simulink model "CP_SFC_Lin_a_n9558292"  (R2018a)
settings: Solver=ode4  StartTime=0.0  StopTime=5  FixedStep=0.02  RelTol=1e-3
values from neighbouring files (symbols this model uses):
  g = 9.81    [CP_SFC_Lin_b_MainFile_n9558292.m]
  l = 0.2    [CP_SFC_Lin_b_MainFile_n9558292.m]
  m = 0.15    [CP_SFC_Lin_b_MainFile_n9558292.m]
  Mc = 0.4    [CP_SFC_Lin_b_MainFile_n9558292.m]
  x10 = 0.4    [CP_SFC_Lin_b_MainFile_n9558292.m]
  x20 = deg2rad(200)    [CP_SFC_Lin_b_MainFile_n9558292.m]
  x30 = 0    [CP_SFC_Lin_b_MainFile_n9558292.m]
  x40 = 0    [CP_SFC_Lin_b_MainFile_n9558292.m]
undefined symbols (not defined in the file or in its folder): Ka
settings Model: Creator=haidarobeid  LastModifiedBy=haidarobeid

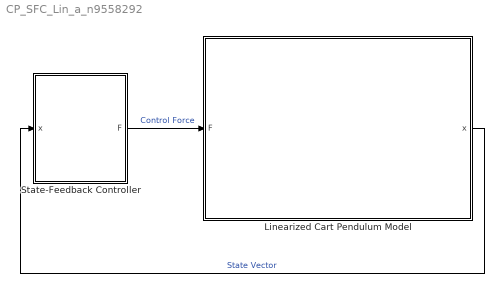
== system CP_SFC_Lin_a_n9558292 ==
  Linearized Cart Pendulum Model : Subsystem
  State-Feedback Controller : Subsystem
  wires:
  State-Feedback Controller/1(F) -> Linearized Cart Pendulum Model/1(F)  "Control Force"
  Linearized Cart Pendulum Model/1(x) -> State-Feedback Controller/1(x)  "State Vector"

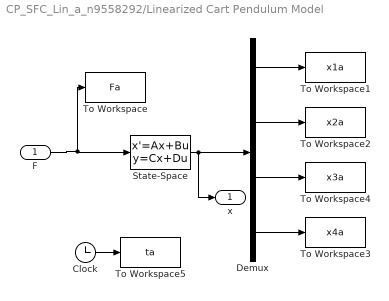
== system CP_SFC_Lin_a_n9558292/Linearized Cart Pendulum Model ==
  F : Inport
  Clock : Clock
  Demux : Demux
  State-Space : StateSpace  A=[0,0,1,0;0,0,0,1;0,-m*g/Mc,0,0;0,g*(Mc+m)/(l*Mc),0,0]  B=[0;0;1/Mc;-1/(l*Mc)]  C=eye(4)  D=[0; 0; 0 ;0]  InitialCondition=[x10;x20;x30;x40]
  To Workspace : ToWorkspace  VariableName=Fa  SampleTime=-1
  To Workspace1 : ToWorkspace  VariableName=x1a  SampleTime=-1
  To Workspace2 : ToWorkspace  VariableName=x2a  SampleTime=-1
  To Workspace3 : ToWorkspace  VariableName=x4a  SampleTime=-1
  To Workspace4 : ToWorkspace  VariableName=x3a  SampleTime=-1
  To Workspace5 : ToWorkspace  VariableName=ta  SampleTime=-1
  x : Outport
  wires:
  Demux/3 -> To Workspace4/1
  Demux/2 -> To Workspace2/1
  Demux/4 -> To Workspace3/1
  State-Space/1 -> Demux/1, x/1
  F/1 -> State-Space/1, To Workspace/1
  Demux/1 -> To Workspace1/1
  Clock/1 -> To Workspace5/1

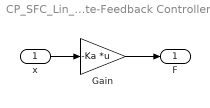
== system CP_SFC_Lin_a_n9558292/State-Feedback Controller ==
  x : Inport
  Gain : Gain  Gain=-Ka  Multiplication=Matrix(K*u)
  F : Outport
  wires:
  Gain/1 -> F/1
  x/1 -> Gain/1
